simulink model "DCMotor"  (R2025a)
settings: Solver=VariableStepAuto  StartTime=0.0  StopTime=15  RelTol=1e-3
undefined symbols (not defined in the file): CGxyz, Gxyz
libraries: nesl_utility x12, fl_lib x10, ee_lib x5, sdl_lib x4, aerolibnav x2
settings Model: SimulationMode=accelerator  Creator=Mazou  LastModifiedBy=Mazou

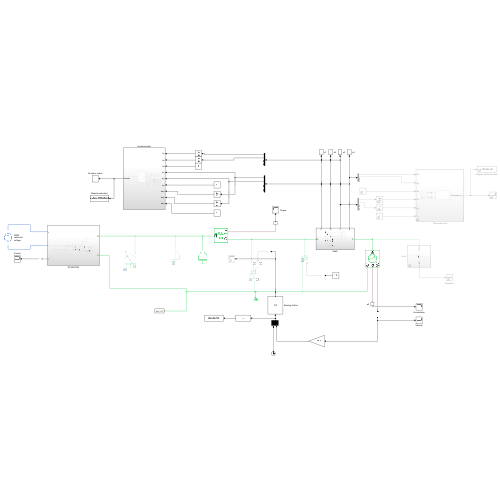
[thumbnail: Simulink's stored preview of the top-level diagram]
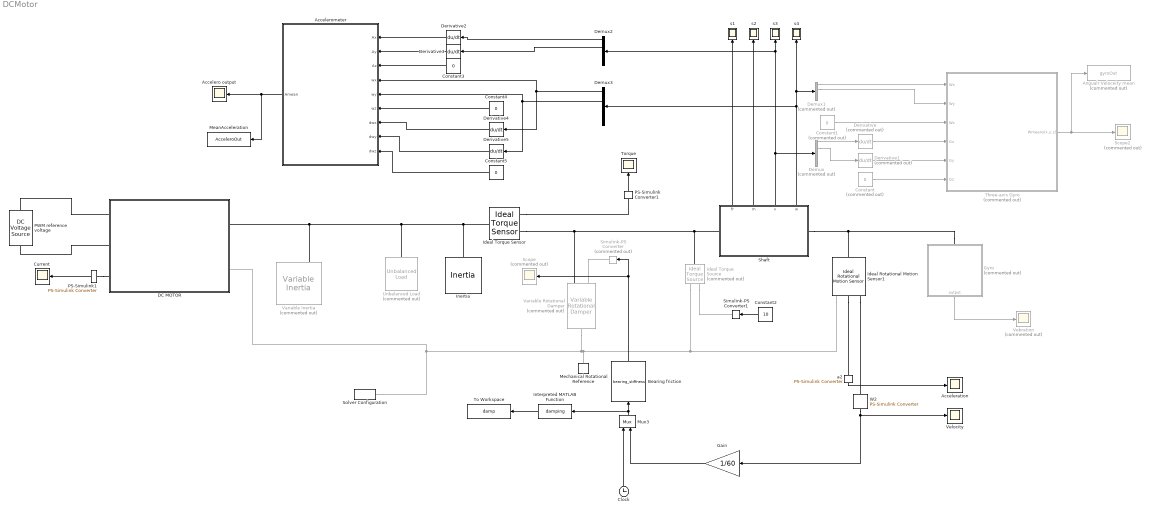
== system DCMotor ==
  Acceleration : Scope
      settings: ActiveDisplayYMinimum=-11.35074  ActiveDisplayYMaximum=102.15664
  Accelero output : Scope
      settings: ActiveDisplayYMinimum=-1.63436  ActiveDisplayYMaximum=11.58913  DataLoggingVariableName=ScopeData5
  Accelerometer : Subsystem
  Angualr Veloceity mean : ToWorkspace  Commented=on  VariableName=gyroOut  SampleTime=-1
      settings: Save2DSignal=2-D array (concatenate along first dimension)
  Bearing friction : MATLABFcn  MATLABFcn=bearing_stiffness
  Clock : Clock
  Constant : Constant  Commented=on  Value=0
  Constant1 : Constant  Commented=on  Value=0
  Constant2 : Constant  Value=10
  Constant3 : Constant  Value=0
  Constant4 : Constant  Value=0
  Constant5 : Constant  Value=0
  Current : Scope
      settings: TimeSpan=10  ActiveDisplayYMinimum=-15.75983  ActiveDisplayYMaximum=141.8385  DataLoggingVariableName=ScopeData2
  DC MOTOR : Subsystem
  Demux : Demux  Commented=on
  Demux1 : Demux  Commented=on
  Demux2 : Demux
  Demux3 : Demux
  Derivative : Derivative  Commented=on
  Derivative1 : Derivative  Commented=on
  Derivative{2..5} (4 alike) : Derivative
  Gain : Gain  Gain=1/60
  Gyro : Subsystem  Commented=on
  Ideal Rotational Motion Sensor1 : fl_lib/Mechanical/Mechanical Sensors/Ideal Rotational Motion Sensor  reference=foundation.enum.MeasurementReference.difference  acceleration_port=true  velocity_port=true  position_port=false  wrap_angle=simscape.enum.onoff.off  offset=0 deg
      settings: LogSimulationData=on  InternalSimscapePortConfiguration="{\"Bottom\":[],\"Left\":[{\"id\":\"R\",\"label\":\"R\",\"type\":\"foundation.mechanical.rotational.rotational\"}],\"Right\":[{\"id\":\"C\",\"label\":\"C\",\"type\":\"foundation.mechanical.rotational.rotational\"},{\"id\":\"alpha\",\"label\":\"α\",\"type\":\"output\"},{\"id\":\"W\",\"label\":\"W\",\"type\":\"output\"}],\"Top\":[]}"
  Ideal Torque Sensor : fl_lib/Mechanical/Mechanical Sensors/Ideal Torque Sensor
      settings: LogSimulationData=on
  Ideal Torque Source : fl_lib/Mechanical/Mechanical Sources/Ideal Torque Source  Commented=on
  Inertia : fl_lib/Mechanical/Rotational Elements/Inertia  inertia=0.0001 kg*m^2  num_ports=foundation.enum.numPorts2.one  w_specify=off  w_priority=High  w=0 rad/s  w_nominal_specify=off  w_nominal_value=1  w_nominal_unit=rad/s  t_specify=off  t_priority=High  t=0 N*m  t_nominal_specify=off  t_nominal_value=1  t_nominal_unit=N*m
      settings: LogSimulationData=on
  Interpreted MATLAB Function : MATLABFcn  MATLABFcn=damping
  MeanAcceleration : ToWorkspace  VariableName=AcceleroOut  SaveFormat=Structure With Time  SampleTime=-1
      settings: Save2DSignal=2-D array (concatenate along first dimension)
  Mechanical Rotational Reference : fl_lib/Mechanical/Rotational Elements/Mechanical Rotational Reference
  Mux3 : Mux  Inputs=2
  PS-Simulink Converter1 : nesl_utility/PS-Simulink Converter  PhysicalDomain=network_engine_domain  SubClassName=ps_output  LeftPortType=input  RightPortType=output  PseudoPeriodic=off  Frequencies=[]  VectorFormat=inherit  Unit=inherit  AffineConversion=off
  PS-Simulink1 : nesl_utility/PS-Simulink Converter  PhysicalDomain=network_engine_domain  SubClassName=ps_output  LeftPortType=input  RightPortType=output  PseudoPeriodic=off  Frequencies=[]  VectorFormat=1-D array  Unit=A  AffineConversion=off
  PWM reference voltage : fl_lib/Electrical/Electrical Sources/DC Voltage Source  v0=2 V
  Scope : Scope  Commented=on
      settings: ActiveDisplayYMinimum=0.0875  ActiveDisplayYMaximum=0.1125
  Scope2 : Scope  Commented=on
      settings: ActiveDisplayYMinimum=-0.10232  ActiveDisplayYMaximum=0.11963  DataLoggingVariableName=ScopeData6
  Shaft : Subsystem
      settings: PortSchema="{\"entries\":[{\"content\":{\"sides\":[{\"content\":{\"connectorIds\":[\"LConn1\"]},\"type\":\"ConnectorPlacement.EquallySpacedRectSide\",\"uuid\":\"3857fe44-01bc-4751-8e4d-1dad1ce500eb\"},{\"content\":{\"connectorIds\":[\"RConn1\"],\"side\":\"RIGHT\"},\"type\":\"ConnectorPlacement.EquallySpacedRectSide\",\"uuid\":\"6a019b46-4414-4623-8f21-6865903b21bc\"},{\"content\":{\"connectorIds\":[\"Out1\",\"Out2\",\"Out3\",\"Out4\"],\"side\":\"TOP\"},\"type\":\"ConnectorPlacement.EquallySpacedRectSide\",\"uuid\":\"f54769ec-328a-48be-bd09-14cbb2038700\"}]},\"type\":\"ConnectorPlacement.EquallySpacedConnector\",\"uuid\":\"c21046b3-6169-4705-a85c-ea50b341e5c4\"}],\"packageUris\":[\"http://schema.mathworks.com/mf0/Connector/R2020b\"],\"version\":\"1.0\"}"
  Simulink-PS Converter : nesl_utility/Simulink-PS Converter  Commented=on  PhysicalDomain=network_engine_domain  SubClassName=ps_input  LeftPortType=input  RightPortType=output  PseudoPeriodic=off  Frequencies=[]  NoiseDistribution=none  NoiseParameters=[]  Unit=1  AffineConversion=off  FilteringAndDerivatives=provide  SimscapeFilterOrder=1  InputFilterTimeConstant=0.001  UdotUserProvided=0
  Simulink-PS Converter1 : nesl_utility/Simulink-PS Converter  PhysicalDomain=network_engine_domain  SubClassName=ps_input  LeftPortType=input  RightPortType=output  PseudoPeriodic=off  Frequencies=[]  NoiseDistribution=none  NoiseParameters=[]  Unit=1  AffineConversion=off  FilteringAndDerivatives=provide  SimscapeFilterOrder=1  InputFilterTimeConstant=0.001  UdotUserProvided=0
  Solver Configuration : nesl_utility/Solver Configuration  PhysicalDomain=network_engine_domain  SubClassName=solver  LeftPortType=input  RightPortType=generic  Tones=[]  Harmonics=[]  SimulateNoise=off  Profile=off  UseLocalSampling=off  EnableSwitchedLinearOptims=on  FrequencyDomain=off  UseCCode=off  RelTol=0.001  AbsTol=1e-06  MinStep=1e-09  ToWorkspace=off  RevertToSquareIcSolve=off  NumHomotopyIterations=100  PhasorMode=off  PhasorModeNumHarmonics=1  ConsistencySolver=NEWTON_FTOL  IndexReductionMethod=DerivativeReplacement  DoDC=off  ResidualTolerance=1e-9  ConsistencyTolSource=GLOBAL  ConsistencyAbsTol=0.001  ConsistencyRelTol=0.001  ConsistencyTolFactor=0.001  UseLocalSolver=off  LocalSolverChoice=NE_BACKWARD_EULER_ADVANCER  ResolveIndetEquations=on  FunctionEvalNumThread=1  LocalSolverSampleTime=5e-6  DoFixedCost=off  MaxNonlinIter=4  MaxModeIter=2  ComputeImpulses=off  ImpulseIterations=2  LinearAlgebra=auto  LinearAlgebraNumThread=0  EquationFormulation=NE_TIME_EF  DelaysMemoryBudget=1024  AutomaticFiltering=on  FilteringTimeConstant=0.001  PartitionStorageMethod=AS_NEEDED  PartitionMemoryBudget=1024  PartitionMethod=FAST  MultibodyUseLocalSolver=off  MultibodyLocalSolverChoice=ODE1  MultibodyLocalSolverSampleTime=0.001
  Three-axis Gyro : Subsystem  Commented=on
  To Workspace : ToWorkspace  VariableName=damp  SampleTime=-1
  Torque : Scope
      settings: ActiveDisplayYMinimum=-0.25583  ActiveDisplayYMaximum=2.30248  DataLoggingVariableName=ScopeData7
  Unbalanced Load : sdl_lib/Inertias & Loads/Unbalanced Load  Commented=on  parameterization=sdl.enum.loadRotation.circular  inertia=0.001 kg*m^2  mass=0.001 kg  r_axis=.50 m  r_rotation=.001 m  r_inline=.01 m  r_perp=.005 m  angle_vector=[0, pi, 3 * pi / 2] rad  inertia_vector=[1, 10, 1] kg*m^2  init_type=sdl.enum.loadInitialization.velocity  init_momentum=0.1 kg*m^2/s  init_vel=0 rad/s  init_angle=0 rad
      settings: InternalSimscapePortConfiguration="{\"Bottom\":[],\"Left\":[{\"id\":\"I\",\"label\":\"\",\"type\":\"foundation.mechanical.rotational.rotational\"}],\"Right\":[],\"Top\":[]}"
  Variable Inertia : sdl_lib/Inertias & Loads/Variable Inertia  Commented=on  minimum_inertia=0.1 g*cm^2  L_specify=off  L_priority=High  L=0 kg*m^2/s  L_nominal_specify=off  L_nominal_value=1  L_nominal_unit=kg*m^2/s
      settings: InternalSimscapePortConfiguration="{\"Bottom\":[],\"Left\":[{\"id\":\"I\",\"label\":\"\",\"type\":\"input\"},{\"id\":\"A\",\"label\":\"\",\"type\":\"foundation.mechanical.rotational.rotational\"}],\"Right\":[],\"Top\":[]}"
  Variable Rotational Damper : sdl_lib/Couplings & Drives/Springs & Dampers/Variable Rotational Damper  Commented=on  Bmin=0 N*m*s/rad
      settings: InternalSimscapePortConfiguration="{\"Bottom\":[],\"Left\":[{\"id\":\"B\",\"label\":\"B\",\"type\":\"input\"},{\"id\":\"R\",\"label\":\"R\",\"type\":\"foundation.mechanical.rotational.rotational\"}],\"Right\":[{\"id\":\"C\",\"label\":\"C\",\"type\":\"foundation.mechanical.rotational.rotational\"}],\"Top\":[]}"
  Vebration : Scope  Commented=on
      settings: ActiveDisplayYMinimum=3.99999999999988  ActiveDisplayYMaximum=4.00000000000009  DataLoggingVariableName=ScopeData8
  Velocity : Scope
      settings: ActiveDisplayYMinimum=1665.13861  ActiveDisplayYMaximum=1706.12975  DataLoggingVariableName=ScopeData2
  W2 : nesl_utility/PS-Simulink Converter  PhysicalDomain=network_engine_domain  SubClassName=ps_output  LeftPortType=input  RightPortType=output  PseudoPeriodic=off  Frequencies=[]  VectorFormat=1-D array  Unit=rpm  AffineConversion=off
  a2 : nesl_utility/PS-Simulink Converter  PhysicalDomain=network_engine_domain  SubClassName=ps_output  LeftPortType=input  RightPortType=output  PseudoPeriodic=off  Frequencies=[]  VectorFormat=inherit  Unit=inherit  AffineConversion=off
  s{1..4} (4 alike) : Scope
      s1 settings: ActiveDisplayYMinimum=-163.69257  ActiveDisplayYMaximum=103.51357  DataLoggingVariableName=ScopeData9
      s2 settings: ActiveDisplayYMinimum=-107.14777  ActiveDisplayYMaximum=107.147  DataLoggingVariableName=ScopeData10
      s3 settings: ActiveDisplayYMinimum=-0.01046  ActiveDisplayYMaximum=0.01046  DataLoggingVariableName=ScopeData11
      s4 settings: ActiveDisplayYMinimum=-0.01718  ActiveDisplayYMaximum=0.01718
  wires:
  Shaft/2(m) -> s2/1
  Derivative5/1 -> Accelerometer/8(dwy)
  Derivative/1 -> Three-axis Gyro/4(Gx)
  Accelerometer/1(Amean) -> Accelero output/1, MeanAcceleration/1
  Clock/1 -> Mux3/1
  PS-Simulink1/1 -> Current/1
  Derivative3/1 -> Accelerometer/2(Ay)
  Demux1/1 -> Three-axis Gyro/1(Wx)
  Gyro/1(output) -> Vebration/1
  Constant5/1 -> Accelerometer/9(dwz)
  PS-Simulink Converter1/1 -> Torque/1
  Demux2/1 -> Derivative2/1
  Derivative4/1 -> Accelerometer/7(dwx)
  Constant3/1 -> Accelerometer/3(Az)
  Demux2/2 -> Derivative3/1
  Constant4/1 -> Accelerometer/6(wz)
  Derivative1/1 -> Three-axis Gyro/5(Gy)
  Shaft/3(v) -> Demux/1, s3/1, Demux2/1
  Three-axis Gyro/1(Wmeans(x,y,z)) -> Scope2/1, Angualr Veloceity mean/1
  Demux/2 -> Derivative1/1
  Constant1/1 -> Three-axis Gyro/3(Wz)
  Demux1/2 -> Three-axis Gyro/2(Wy)
  Constant/1 -> Three-axis Gyro/6(Gz)
  Shaft/1(fr) -> s1/1
  a2/1 -> Acceleration/1
  Demux3/2 -> Derivative5/1, Accelerometer/5(wy)
  Demux/1 -> Derivative/1
  W2/1 -> Velocity/1, Gain/1
  Gain/1 -> Mux3/2
  Demux3/1 -> Derivative4/1, Accelerometer/4(wx)
  Derivative2/1 -> Accelerometer/1(Ax)
  Shaft/4(w) -> Demux3/1, s4/1, Demux1/1
  Mux3/1 -> Bearing friction/1, Interpreted MATLAB Function/1
  Constant2/1 -> Simulink-PS Converter1/1
  Bearing friction/1 -> Scope/1, Simulink-PS Converter/1
  Interpreted MATLAB Function/1 -> To Workspace/1
  connections:
  Variable Rotational Damper/RConn1 -- Solver Configuration/RConn1 -- DC MOTOR/RConn2 -- Ideal Rotational Motion Sensor1/RConn1 -- Ideal Torque Source/RConn2 -- Mechanical Rotational Reference/LConn1
  Gyro/LConn1 -- Shaft/RConn1 -- Ideal Rotational Motion Sensor1/LConn1
  Ideal Rotational Motion Sensor1/RConn3 -- W2/LConn1
  DC MOTOR/LConn2 -- PWM reference voltage/RConn1
  Ideal Rotational Motion Sensor1/RConn2 -- a2/LConn1
  Simulink-PS Converter/RConn1 -- Variable Rotational Damper/LConn1
  PWM reference voltage/LConn1 -- DC MOTOR/LConn1
  Ideal Torque Source/RConn1 -- Simulink-PS Converter1/RConn1
  PS-Simulink1/LConn1 -- DC MOTOR/LConn3
  Ideal Torque Sensor/RConn2 -- PS-Simulink Converter1/LConn1
  Shaft/LConn1 -- Ideal Torque Sensor/RConn1 -- Variable Rotational Damper/LConn2 -- Ideal Torque Source/LConn1
  Ideal Torque Sensor/LConn1 -- Unbalanced Load/LConn1 -- DC MOTOR/RConn1 -- Variable Inertia/LConn2 -- Inertia/LConn1

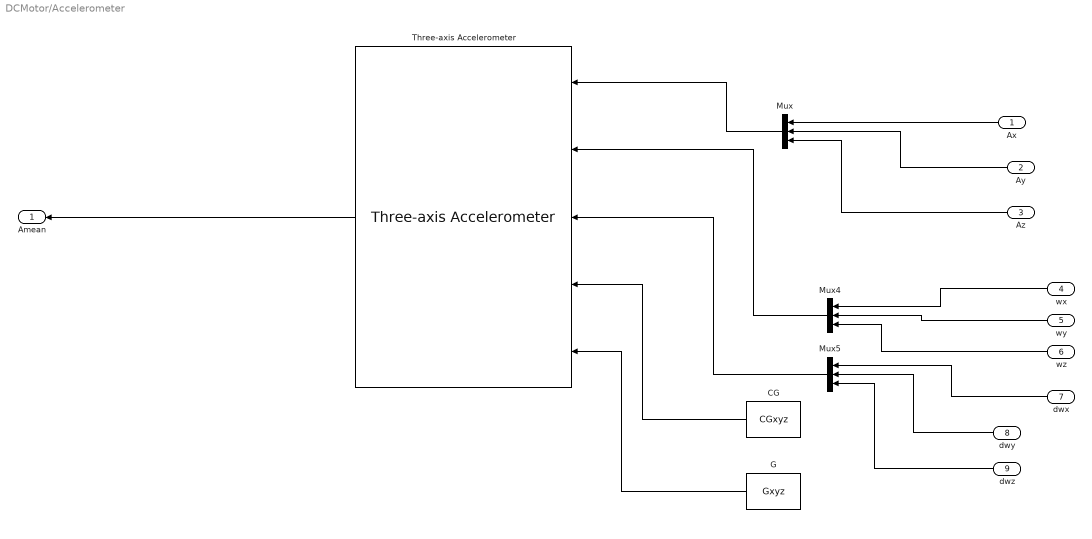
== system DCMotor/Accelerometer ==
  Ax : Inport
  Ay : Inport  Port=2
  Az : Inport  Port=3
  wx : Inport  Port=4
  wy : Inport  Port=5
  wz : Inport  Port=6
  dwx : Inport  Port=7
  dwy : Inport  Port=8
  dwz : Inport  Port=9
  CG : Constant  Value=CGxyz
  G : Constant  Value=Gxyz
  Mux : Mux  Inputs=3
  Mux4 : Mux  Inputs=3
  Mux5 : Mux  Inputs=3
  Three-axis Accelerometer : aerolibnav/Three-axis Accelerometer  units=Metric (MKS)  acc=[0 0 0]  gtype=on  dtype_a=on  w_a=190  z_a=0.707  a_sf_cc=[1 0 0; 0 1 0; 0 0 1]  a_bias=[0 0 0]  a_Ts=0  a_rand=on  a_seeds=[23093 23094 23095]  a_pow=[0.001 0.001 0.001]  a_sat="[-inf  -inf  -inf  inf inf inf]"
  Amean : Outport
  wires:
  CG/1 -> Three-axis Accelerometer/4
  Mux4/1 -> Three-axis Accelerometer/2
  wy/1 -> Mux4/2
  Mux/1 -> Three-axis Accelerometer/1
  G/1 -> Three-axis Accelerometer/5
  Az/1 -> Mux/3
  Three-axis Accelerometer/1 -> Amean/1
  Mux5/1 -> Three-axis Accelerometer/3
  dwy/1 -> Mux5/2
  dwx/1 -> Mux5/1
  Ax/1 -> Mux/1
  wx/1 -> Mux4/1
  dwz/1 -> Mux5/3
  wz/1 -> Mux4/3
  Ay/1 -> Mux/2

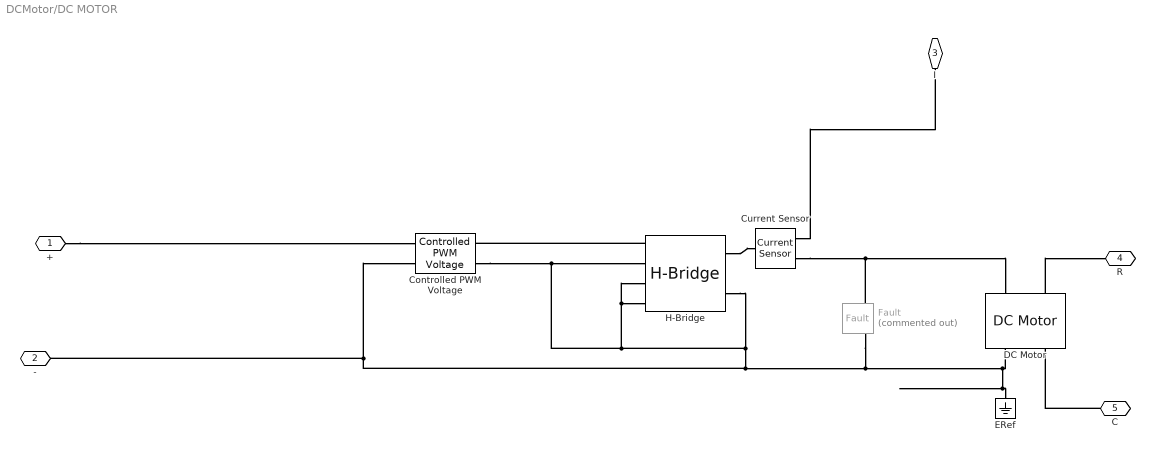
== system DCMotor/DC MOTOR ==
  Controlled PWM Voltage : ee_lib/Integrated Circuits/Controlled PWM Voltage  F=4000 Hz  TD=0 s  pulse_width_offset=0 s  pulse_min=0 s  pwm_or_av=2  event_type=1  sample_time=5e-6 s  Vmin=0 V  Vmax=5 V  Vm=5 V  u_min=0  u_max=1
  Current Sensor : fl_lib/Electrical/Electrical Sensors/Current Sensor
  DC Motor : ee_lib/Electromechanical/Brushed Motors/DC Motor  PartSpecification="{\"DatasetId\":\"Maxon|RE_65_388985_24|simscape.electrical.dcMotor\",\"DisplayName\":\"Maxon:RE_65_388985_24\"}"  field_option=ee.enum.field_option.pm  Rf=100 % Parameter not set Ohm  Lf=1 % Parameter not set H  Laf=0.15 % Parameter not set H  If0=0 % Parameter not set A  parameterization=ee.enum.dcparam_option.circuit_param  Ra=0.0891 % Datasheet derived Ohm  La=0.031 % Datasheet derived mH  emf_or_torque=ee.enum.emf_or_torque.ki  Kv=5.62345 % Parameter estimated mV/rpm  Ki=53.7 % Datasheet derived mN*m/A  T_stall=0.24e-3 % Parameter not set N*m  w_max=19100 % Parameter not set rpm  w_rated=15000 % Parameter not set rpm  P_rated=0.08 % Parameter not set W  V_rated=1.5 % Parameter not set V  lam_param=ee.enum.lam_param.current  i_noload=0.697 % Datasheet derived A  V_i_noload=24 % Datasheet derived V  J=1200 g*cm^2  lam=0 % % Parameter not set mN*m/(rad/s)  speed0=0.0% Parameter not set rad/s  alpha=3.93e-3 % Parameter not set 1/K  Tmeas=25 % Parameter not set degC  thermal_mass=667.588357588358 % Parameter estimated J/K  initial_temperature=25 % Parameter not set degC
      settings: AttributesFormatString=Maxon:RE_65_388985_24
  ERef : fl_lib/Electrical/Electrical Elements/Electrical Reference
  Fault : ee_lib/Utilities/Fault  Commented=on  R_unfaulted=inf Ohm  R_faulted=1e-3 Ohm  fault_action=1  enable_temporal_fault=0  t_fault=5 s  fault_duration=inf s  enable_behavioral_fault=0  permissible_voltage_range=[-100, 100] V  t_fail_on_voltage=1 s  permissible_current_range=[-1, 1] A  t_fail_on_current=1 s  enable_external_fault=0  fault_condition=1  fault_threshold=0.5  fault_resettable=0
      settings: InternalSimscapePortConfiguration="{\"Bottom\":[],\"Left\":[{\"id\":\"p\",\"label\":\"+\",\"type\":\"foundation.electrical.electrical\"},{\"id\":\"F\",\"label\":\"F\",\"type\":\"input\"}],\"Right\":[{\"id\":\"n\",\"label\":\"-\",\"type\":\"foundation.electrical.electrical\"},{\"id\":\"X\",\"label\":\"X\",\"type\":\"output\"}],\"Top\":[]}"
  H-Bridge : ee_lib/Semiconductors & Converters/Converters/H-Bridge  supply_ports=ee.enum.supply_ports.hidesupply  pwm_or_av=2  regenerative_braking_mode=2  discontinuous=0  freewheeling_mode=1  Rload=3.38+0.1 Ohm  Lload=1e-5 H  F=4 kHz  Venable=2.5 V  Vmax=5 V  Vreverse=2.5 V  Vbrake=2.5 V  Vm=24 V  Ron=0.1 Ohm  Don=0.1 Ohm  Goff=1e-6 S  Tmeas=298.15 K  Ron2=0.1 Ohm  Don2=0.05 Ohm  Tmeas2=398.15 K  thermal_mass=100 J/K  initial_temperature=298.15 K
  + : PMIOPort  Side=Left
  - : PMIOPort  Port=2  Side=Left
  I : PMIOPort  Port=3  Side=Left
  R : PMIOPort  Port=4  Side=Right
  C : PMIOPort  Port=5  Side=Right
  connections:
  H-Bridge/LConn1 -- Controlled PWM Voltage/RConn1
  Current Sensor/RConn2 -- Fault/LConn1 -- DC Motor/LConn1
  -/RConn1 -- Controlled PWM Voltage/LConn2 -- H-Bridge/RConn2 -- H-Bridge/LConn3 -- H-Bridge/LConn4 -- H-Bridge/LConn2 -- Controlled PWM Voltage/RConn2 -- Fault/RConn1 -- DC Motor/RConn1 -- ERef/LConn1
  +/RConn1 -- Controlled PWM Voltage/LConn1
  H-Bridge/RConn1 -- Current Sensor/LConn1
  Current Sensor/RConn1 -- I/RConn1
  C/RConn1 -- DC Motor/RConn2
  DC Motor/LConn2 -- R/RConn1

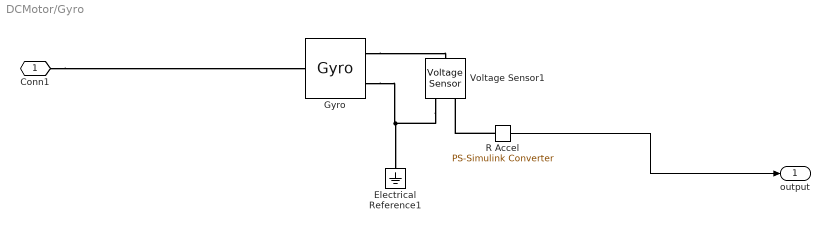
== system DCMotor/Gyro ==
  Electrical Reference1 : fl_lib/Electrical/Electrical Elements/Electrical Reference
  Gyro : ee_lib/Sensors & Transducers/Gyro  sensitivity=12.5 mV*s/deg  v_null=2.5 V  v_max=4 V  v_min=1 V  model_dynamics=0  bw=3 kHz  w_meas_specify=off  w_meas_priority=Low  w_meas=0 deg/s  w_meas_nominal_specify=off  w_meas_nominal_value=1  w_meas_nominal_unit=deg/s
      settings: InternalSimscapePortConfiguration="{\"Bottom\":[],\"Left\":[{\"id\":\"R\",\"label\":\"R\",\"type\":\"foundation.mechanical.rotational.rotational\"}],\"Right\":[{\"id\":\"p\",\"label\":\"+\",\"type\":\"foundation.electrical.electrical\"},{\"id\":\"n\",\"label\":\"-\",\"type\":\"foundation.electrical.electrical\"}],\"Top\":[]}"
  R Accel : nesl_utility/PS-Simulink Converter  PhysicalDomain=network_engine_domain  SubClassName=ps_output  LeftPortType=input  RightPortType=output  PseudoPeriodic=off  Frequencies=[]  VectorFormat=inherit  Unit=inherit  AffineConversion=off
  Voltage Sensor1 : fl_lib/Electrical/Electrical Sensors/Voltage Sensor
  Conn1 : PMIOPort  Side=Left
  output : Outport
  wires:
  R Accel/1 -> output/1
  connections:
  R Accel/LConn1 -- Voltage Sensor1/RConn1
  Conn1/RConn1 -- Gyro/LConn1
  Gyro/RConn1 -- Voltage Sensor1/LConn1
  Voltage Sensor1/RConn2 -- Gyro/RConn2 -- Electrical Reference1/LConn1

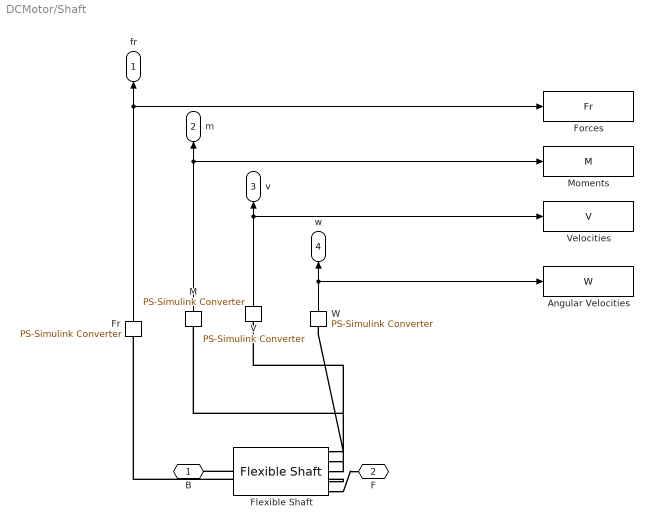
== system DCMotor/Shaft ==
  Angular Velocities : ToWorkspace  VariableName=W  SampleTime=-1
      settings: Save2DSignal=2-D array (concatenate along first dimension)
  Flexible Shaft : sdl_lib/Couplings & Drives/Flexible Shaft  modelTorsion=false  modelTransverse=true  n_segments=1  parameterization=sdl.enum.shaftParameterization.StiffnessInertia  length=1 m  lengths=[1, .5, .25] m  shaft_stiffness=2e5 N*m/rad  shaft_inertia=0.02 kg*m^2  shaft_stiffnesses=[400000, 200000, 100000] N*m/rad  shaft_inertias=[.025, .02, .015] kg*m^2  eiIN=5e5 Pa*m^4  rhoaIN=19 kg/m  eiINs=[600000, 500000, 400000] Pa*m^4  rhoaINs=[20, 19, 18] kg/m  density=7.8e3 kg/m^3  shear_modulus=7.93e9 Pa  elastic_modulus=200e9 Pa  shaft_construction=sdl.enum.shaftConstruction.solid  diameter_outer=0.075 m  diameter_inner=0.05 m  diameter_outers=[.085, .075, .065] m  diameter_inners=[.055, .05, .045] m  damping_ratio=0.01  mu_visc_BF=[0, 0] N*m*s/rad  mu_visc=[0, 0] N*m*s/rad  initial_deflection=0 rad  initial_velocity=0 rpm  num_supports=sdl.enum.num_supports.two  z_support=[0, 1] m  boundaryB1=sdl.enum.shaftSupport.bearingMatrix  DrotB1_row=[1000, 1000] N*m*s/rad  DtransB1_row=[20000, -44000, -44000, 350000] N*s/m  DtransB1_w_mat=[20000, -44000, -44000, 350000; 10000, -25000, -25000, 140000; 5000, -10000, -10000, 20000] N*s/m  KrotB1_row=[10000, 10000] N*m/rad  KtransB1_row=[1000000, -200000, -300000, 5000000] N/m  KtransB1_w_mat=[1000000, -600000, -3500000, 8000000; 1000000, -200000, -3000000, 5000000; 1000000, -50000, -2500000, 3000000] N/m  boundaryI1=sdl.enum.shaftSupport.clamp  DrotI1_row=[1000, 1000] N*m*s/rad  DtransI1_row=[20000, -44000, -44000, 350000] N*s/m  DtransI1_w_mat=[20000, -44000, -44000, 350000; 10000, -25000, -25000, 140000; 5000, -10000, -10000, 20000] N*s/m  KrotI1_row=[10000, 10000] N*m/rad  KtransI1_row=[1000000, -200000, -300000, 5000000] N/m  KtransI1_w_mat=[1000000, -600000, -3500000, 8000000; 1000000, -200000, -3000000, 5000000; 1000000, -50000, -2500000, 3000000] N/m  boundaryI2=sdl.enum.shaftSupport.clamp  DrotI2_row=[1000, 1000] N*m*s/rad  DtransI2_row=[20000, -44000, -44000, 350000] N*s/m  DtransI2_w_mat=[20000, -44000, -44000, 350000; 10000, -25000, -25000, 140000; 5000, -10000, -10000, 20000] N*s/m  KrotI2_row=[10000, 10000] N*m/rad  KtransI2_row=[1000000, -200000, -300000, 5000000] N/m  KtransI2_w_mat=[1000000, -600000, -3500000, 8000000; 1000000, -200000, -3000000, 5000000; 1000000, -50000, -2500000, 3000000] N/m  boundaryF1=sdl.enum.shaftSupport.clamp  DrotF1_row=[1000, 1000] N*m*s/rad  DtransF1_row=[20000, -44000, -44000, 350000] N*s/m  DtransF1_w_mat=[20000, -44000, -44000, 350000; 10000, -25000, -25000, 140000; 5000, -10000, -10000, 20000] N*s/m  KrotF1_row=[10000, 10000] N*m/rad  KtransF1_row=[1000000, -200000, -300000, 5000000] N/m  KtransF1_w_mat=[1000000, -600000, -3500000, 8000000; 1000000, -200000, -3000000, 5000000; 1000000, -50000, -2500000, 3000000] N/m  bearing_speed=[200, 500, 1500] rpm  alpha=10 1/s  beta=1e-8 s  noDisk=sdl.enum.shaftDisks.none  zDisk=0.5 m  mDiskIN=2 kg  IdDiskIN=0.025 kg*m^2  IpDiskIN=0.050 kg*m^2  enable_static_unbalance=true  offsetMR=[.001, .001] kg*m  offsetMR_initialAngleIN=[0, pi] deg  offsetMassLocation=[.33, .67] m  enable_external_force=false  externalForce=[1, 2] N  externalForceHarmonic=[.5, 2]  externalLoadAngle=[pi / 2, 3 * pi / 4] rad  zExternalLoad=[.25, .75] m  AnalysisMethod=sdl.enum.bendingAnalysisMethod.LumpedMass  ModeInputMethod=sdl.enum.modeInputMethod.SimscapeDetermined  numModesIn=6  mode_speed_dependency=sdl.enum.mode_speed_dependency.Static  OmegaNom=5000 rpm  wMax=1e8 rpm  dz=0.01 m  userMode_w=[280, 644, 615, 1285] rad/s  userMode_w_mat=[257, 780, 580, 1560; 280, 644, 615, 1285; 294, 513, 636, 1020] rad/s  userMode_z=[0, .1, .2, .3, .4, .5, .6, .7, .8, .9, 1] m  userMode_shapeX=[.1648, .0086, -.2759, .0162; .1671, .0093, -.2231, .0133; .1691, .01, -.1689, .0102; .1707, .0105, -.1135, .007; .1717, .0108, -.057, .0035; .1721, .0109, 0, 0; .1717, .0108, .057, -.0035; .1707, .0105, .1135, -.007; .1691, .01, .1689, -.0102; .1671, .0093, .2231, -.0133; .1648, .0086, .2759, -.0162]  userMode_shapeX_mat=cat(3, [.1842, .0134, -.3072, .0272; .1863, .0152, -.2482, .0226; .1882, .0169, -.1878, .0176; .1897, .0182, -.1261, .0121; .1906, .019, -.0634, .0062; .191, .0193, 0, 0; .1906, .019, .0634, -.0062; .1897, .0182, .1261, -.0121; .1882, .0169, .1878, -.0176; .1863, .0152, .2482, -.0226; .1842, .0134, .3072, -.0272], [.1648, .0086, -.2759, .0162; .1671, .0093, -.2231, .0133; .1691, .01, -.1689, .0102; .1707, .0105, -.1135, .007; .1717, .0108, -.057, .0035; .1721, .0109, 0, 0; .1717, .0108, .057, -.0035; .1707, .0105, .1135, -.007; .1691, .01, .1689, -.0102; .1671, .0093, .2231, -.0133; .1648, .0086, .2759, -.0162], [.1291, .0046, -.2166, .0082; .131, .0048, -.1751, .0067; .1327, .005, -.1327, .0051; .1341, .0052, -.0891, .0035; .135, .0053, -.0448, .0017; .1353, .0053, 0, 0; .135, .0053, .0448, -.0017; .1341, .0052, .0891, -.0035; .1327, .005, .1327, -.0051; .131, .0048, .1751, -.0067; .1291, .0046, .2166, -.0082])  userMode_shapeY=[.1193, -.1784, -.1997, -.3348; .1209, -.1933, -.1615, -.2751; .1224, -.2068, -.1223, -.2119; .1235, -.2176, -.0821, -.1445; .1243, -.2245, -.0413, -.0734; .1246, -.2269, 0, 0; .1243, -.2245, .0413, .0734; .1235, -.2176, .0821, .1445; .1224, -.2068, .1223, .2119; .1209, -.1933, .1615, .2751; .1193, -.1784, .1997, .3348]  userMode_shapeY_mat=cat(3, [.0885, -.1625, -.1475, -.3301; .0895, -.1847, -.1192, -.2745; .0904, -.2048, -.0902, -.2141; .0911, -.2209, -.0606, -.1475; .0916, -.2313, -.0304, -.0754; .0917, -.2349, 0, 0; .0916, -.2313, .0304, .0754; .0911, -.2209, .0606, .1475; .0904, -.2048, .0902, .2141; .0895, -.1847, .1192, .2745; .0885, -.1625, .1475, .3301], [.1193, -.1784, -.1997, -.3348; .1209, -.1933, -.1615, -.2751; .1224, -.2068, -.1223, -.2119; .1235, -.2176, -.0821, -.1445; .1243, -.2245, -.0413, -.0734; .1246, -.2269, 0, 0; .1243, -.2245, .0413, .0734; .1235, -.2176, .0821, .1445; .1224, -.2068, .1223, .2119; .1209, -.1933, .1615, .2751; .1193, -.1784, .1997, .3348], [.1566, -.1901, -.2628, -.3377; .1589, -.1994, -.2125, -.2753; .161, -.2079, -.1609, -.2103; .1627, -.2146, -.1081, -.1424; .1638, -.219, -.0544, -.0719; .1642, -.2205, 0, 0; .1638, -.219, .0544, .0719; .1627, -.2146, .1081, .1424; .161, -.2079, .1609, .2103; .1589, -.1994, .2125, .2753; .1566, -.1901, .2628, .3377])  eta_lumped_nominal=1  etaDer_lumped_nominal=1  eta_modal_nominal=1  etaDer_modal_nominal=1
      settings: InternalSimscapePortConfiguration="{\"Bottom\":[{\"id\":\"Fsupports\",\"label\":\"Fr\",\"type\":\"output\"},{\"id\":\"Msupports\",\"label\":\"M\",\"type\":\"output\"},{\"id\":\"Vsupports\",\"label\":\"V\",\"type\":\"output\"},{\"id\":\"Wsupports\",\"label\":\"W\",\"type\":\"output\"}],\"Left\":[{\"id\":\"B\",\"label\":\"B\",\"type\":\"foundation.mechanical.rotational.rotational\"}],\"Right\":[{\"id\":\"F\",\"label\":\"F\",\"type\":\"foundation.mechanical.rotational.rotational\"}],\"Top\":[]}"
  Forces : ToWorkspace  VariableName=Fr  SampleTime=-1
      settings: Save2DSignal=2-D array (concatenate along first dimension)
  Fr : nesl_utility/PS-Simulink Converter  PhysicalDomain=network_engine_domain  SubClassName=ps_output  LeftPortType=input  RightPortType=output  PseudoPeriodic=off  Frequencies=[]  VectorFormat=inherit  Unit=inherit  AffineConversion=off
  M : nesl_utility/PS-Simulink Converter  PhysicalDomain=network_engine_domain  SubClassName=ps_output  LeftPortType=input  RightPortType=output  PseudoPeriodic=off  Frequencies=[]  VectorFormat=inherit  Unit=inherit  AffineConversion=off
  Moments : ToWorkspace  VariableName=M  SampleTime=-1
      settings: Save2DSignal=2-D array (concatenate along first dimension)
  V : nesl_utility/PS-Simulink Converter  PhysicalDomain=network_engine_domain  SubClassName=ps_output  LeftPortType=input  RightPortType=output  PseudoPeriodic=off  Frequencies=[]  VectorFormat=inherit  Unit=inherit  AffineConversion=off
  Velocities : ToWorkspace  VariableName=V  SampleTime=-1
      settings: Save2DSignal=2-D array (concatenate along first dimension)
  W : nesl_utility/PS-Simulink Converter  PhysicalDomain=network_engine_domain  SubClassName=ps_output  LeftPortType=input  RightPortType=output  PseudoPeriodic=off  Frequencies=[]  VectorFormat=inherit  Unit=inherit  AffineConversion=off
  B : PMIOPort  Side=Left
  F : PMIOPort  Port=2  Side=Right
  fr : Outport
  m : Outport  Port=2
  v : Outport  Port=3
  w : Outport  Port=4
  wires:
  M/1 -> Moments/1, m/1
  V/1 -> v/1, Velocities/1
  W/1 -> w/1, Angular Velocities/1
  Fr/1 -> fr/1, Forces/1
  connections:
  Flexible Shaft/RConn5 -- W/LConn1
  Flexible Shaft/RConn2 -- Fr/LConn1
  Flexible Shaft/RConn4 -- V/LConn1
  Flexible Shaft/RConn3 -- M/LConn1
  Flexible Shaft/LConn1 -- B/RConn1
  Flexible Shaft/RConn1 -- F/RConn1

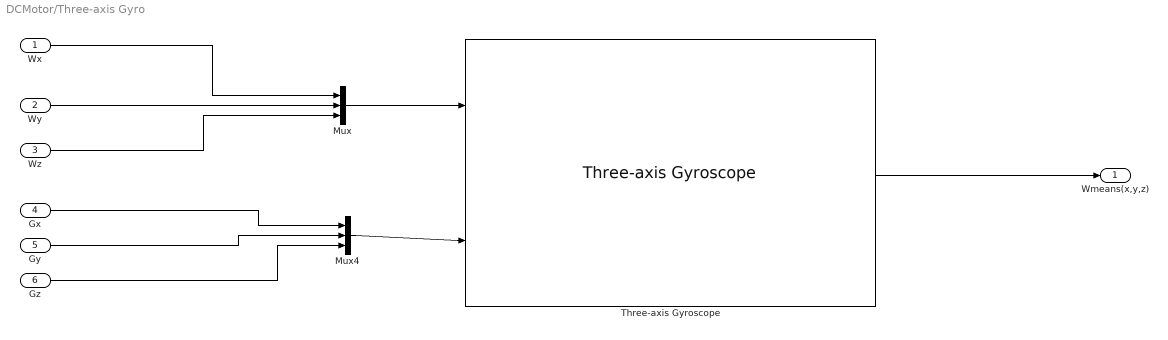
== system DCMotor/Three-axis Gyro ==
  Wx : Inport
  Wy : Inport  Port=2
  Wz : Inport  Port=3
  Gx : Inport  Port=4
  Gy : Inport  Port=5
  Gz : Inport  Port=6
  Mux : Mux  Inputs=3
  Mux4 : Mux  Inputs=3
  Three-axis Gyroscope : aerolibnav/Three-axis Gyroscope  dtype_g=on  w_g=190  z_g=0.707  g_sf_cc=[1 0 0; 0 1 0; 0 0 1]  g_bias=[0 0 0]  g_sen=[0 0 0]  g_Ts=0  g_rand=on  g_seeds=[23093 23094 23095]  g_pow=[0.0001 0.0001 0.0001]  g_sat="[-inf  -inf  -inf  inf inf inf]"
  Wmeans(x,y,z) : Outport
  wires:
  Wz/1 -> Mux/3
  Mux/1 -> Three-axis Gyroscope/1
  Wx/1 -> Mux/1
  Mux4/1 -> Three-axis Gyroscope/2
  Three-axis Gyroscope/1 -> Wmeans(x,y,z)/1
  Gx/1 -> Mux4/1
  Gz/1 -> Mux4/3
  Wy/1 -> Mux/2
  Gy/1 -> Mux4/2
